simulink model "FinalProject_F24_thruster"  (R2023b)
settings: Solver=VariableStepAuto  StartTime=0.0  StopTime=720  FixedStep=.1  MaxStep=0.1  RelTol=1e-3
values from neighbouring files (symbols this model uses):
  h1 = I_s*ws1    [FinalProject_nonlinear_LVLH.m]
  h2 = I_s*ws2    [FinalProject_nonlinear_LVLH.m]
  h3 = I_s*ws3    [FinalProject_nonlinear_LVLH.m]
  hw_0 = [h1;h2;h3]    [FinalProject_nonlinear_LVLH.m]
  I_s =     [FinalProject_nonlinear_LVLH.m]
  I_T = diag([Ir;Ip;Iy])    [FinalProject_nonlinear_LVLH.m]
  K = lqr(A,B,Q,R)    [FinalProject_nonlinear_LVLH.m]
  omega_0 = [0;0;0]    [FinalProject_nonlinear_LVLH.m]
  omega_c = sqrt(mu/a^3)    [FinalProject_nonlinear_LVLH.m]
  q_0 = angle2quat(phi,theta,psi,'XYZ')'    [FinalProject_nonlinear_LVLH.m]
undefined symbols (not defined in the file or in its folder): E_des
libraries: sharedtransform x2
settings Model: Creator=Nathan.Collins  LastModifiedBy=Connor Emmons
settings OptimizationCC: ReuseModelBlockBuffer=off

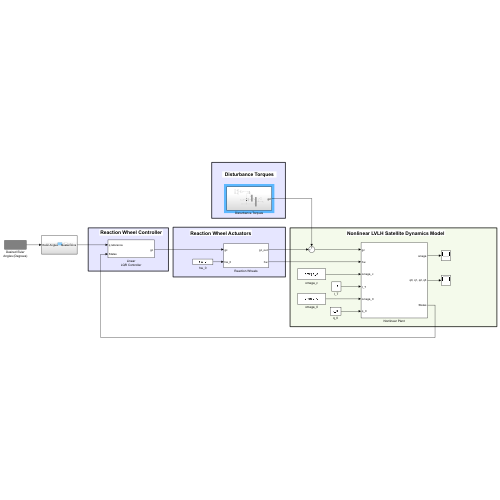
[thumbnail: Simulink's stored preview of the top-level diagram]
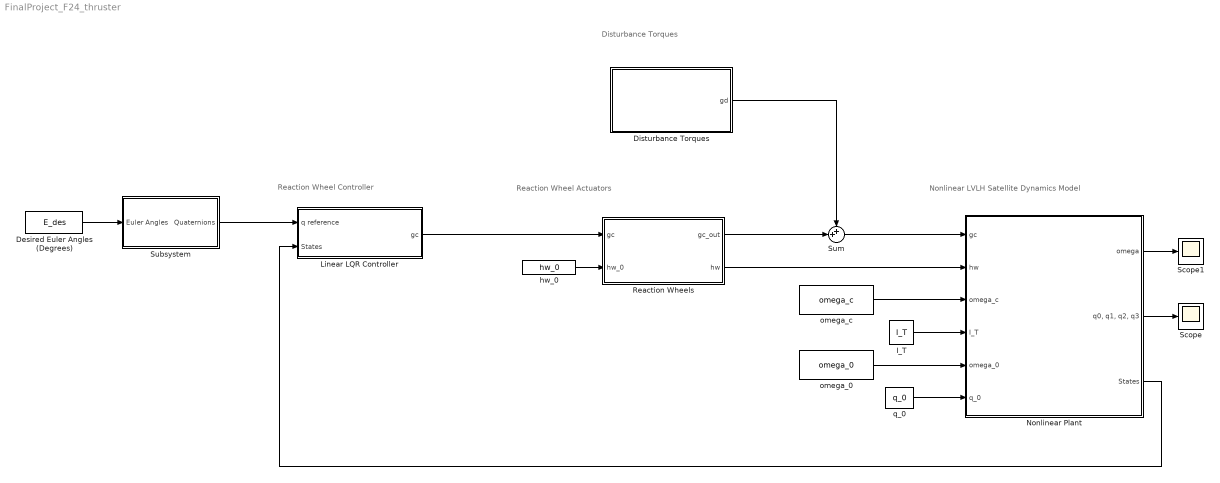
== system FinalProject_F24_thruster ==
  note: Reaction Wheel Actuators
  note: Nonlinear LVLH Satellite Dynamics Model
  note: Reaction Wheel Controller
  note: Disturbance Torques
  Desired Euler Angles (Degrees) : Constant  Value=E_des
  Disturbance Torques : Subsystem
  I_T : Constant  Value=I_T
  Linear LQR Controller : Subsystem
      settings: PortSchema="{\"entries\":[{\"content\":{\"sides\":[{\"content\":{\"connectorIds\":[\"Out1\"]},\"type\":\"ConnectorPlacement.EquallySpacedRectSide\",\"uuid\":\"ee26b0f2-a486-452c-b447-e59bb95ac0cf\"},{\"content\":{\"connectorIds\":[\"In1\",\"In2\"],\"side\":\"RIGHT\"},\"type\":\"ConnectorPlacement.EquallySpacedRectSide\",\"uuid\":\"56766a12-bb91-439a-8915-7afd5112c149\"},{\"content\":{\"connectorIds\":[],\"side\":\"TOP\"},\"type\":\"ConnectorPlacement.EquallySpacedRectSide\",\"uuid\":\"db65a026-f15d-443c-9f95-6ab7980aa8cf\"}]},\"type\":\"ConnectorPlacement.EquallySpacedConnector\",\"uuid\":\"3d1a91a6-4ad3-4b3e-bae7-10d191a9ffc1\"}],\"packageUris\":[\"http://schema.mathworks.com/mf0/Connector/R2020b\"],\"version\":\"1.0\"}"
  Nonlinear Plant : Subsystem
  Reaction Wheels : Subsystem
  Scope : Scope
  Scope1 : Scope
  Subsystem : Subsystem
  Sum : Sum  Inputs=++|
  hw_0 : Constant  Value=hw_0
  omega_0 : Constant  Value=omega_0
  omega_c : Constant  Value=omega_c
  q_0 : Constant  Value=q_0
  wires:
  Reaction Wheels/1(gc_out) -> Sum/2
  Reaction Wheels/2(hw) -> Nonlinear Plant/2(hw)
  omega_c/1 -> Nonlinear Plant/3(omega_c)
  I_T/1 -> Nonlinear Plant/4(I_T)
  hw_0/1 -> Reaction Wheels/2(hw_0)
  omega_0/1 -> Nonlinear Plant/5(omega_0)
  q_0/1 -> Nonlinear Plant/6(q_0)
  Linear LQR Controller/1(gc) -> Reaction Wheels/1(gc)
  Sum/1 -> Nonlinear Plant/1(gc)
  Disturbance Torques/1(gd) -> Sum/1
  Nonlinear Plant/2("q0, q1, q2, q3") -> Scope/1
  Nonlinear Plant/1(omega) -> Scope1/1
  Nonlinear Plant/3(States) -> Linear LQR Controller/2(States)
  Desired Euler Angles (Degrees)/1 -> Subsystem/1(Euler Angles)
  Subsystem/1(Quaternions) -> Linear LQR Controller/1(q reference)

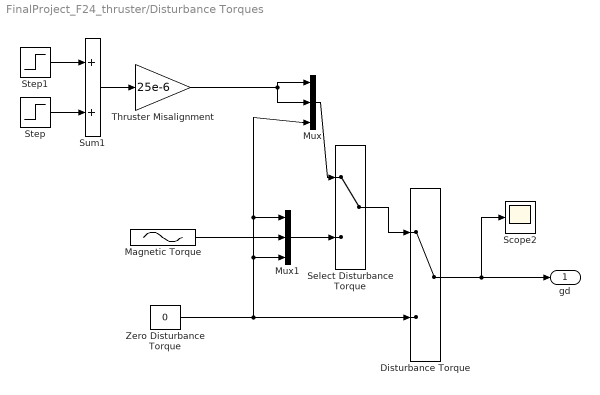
== system FinalProject_F24_thruster/Disturbance Torques ==
  Disturbance Torque : ManualSwitch
  Magnetic Torque : Sin  Amplitude=2e-6  Frequency=2*omega_c  SampleTime=0
  Mux : Mux  Inputs=3
  Mux1 : Mux  Inputs=3
  Scope2 : Scope
  Select Disturbance Torque : ManualSwitch
  Step : Step  Time=300  After=-1  SampleTime=0
  Step1 : Step  Time=0  SampleTime=0
  Sum1 : Sum
  Thruster Misalignment : Gain  Gain=25e-6
  Zero Disturbance Torque : Constant  Value=0
  gd : Outport
  wires:
  Thruster Misalignment/1 -> Mux/2, Mux/1
  Mux/1 -> Select Disturbance Torque/1
  Step1/1 -> Sum1/1
  Sum1/1 -> Thruster Misalignment/1
  Disturbance Torque/1 -> gd/1, Scope2/1
  Step/1 -> Sum1/2
  Zero Disturbance Torque/1 -> Mux/3, Mux1/1, Mux1/3, Disturbance Torque/2
  Mux1/1 -> Select Disturbance Torque/2
  Magnetic Torque/1 -> Mux1/2
  Select Disturbance Torque/1 -> Disturbance Torque/1

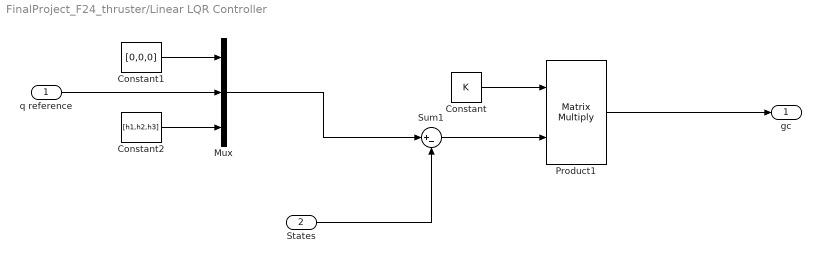
== system FinalProject_F24_thruster/Linear LQR Controller ==
  q reference : Inport
  States : Inport  Port=2
  Constant : Constant  Value=K
  Constant1 : Constant  Value=[0,0,0]
  Constant2 : Constant  Value=[h1,h2,h3]
  Mux : Mux  Inputs=3
  Product1 : Product  Multiplication=Matrix(*)
  Sum1 : Sum  Inputs=|+-
  gc : Outport
  wires:
  States/1 -> Sum1/2
  Product1/1 -> gc/1
  q reference/1 -> Mux/2
  Sum1/1 -> Product1/2
  Constant/1 -> Product1/1
  Constant1/1 -> Mux/1
  Mux/1 -> Sum1/1
  Constant2/1 -> Mux/3

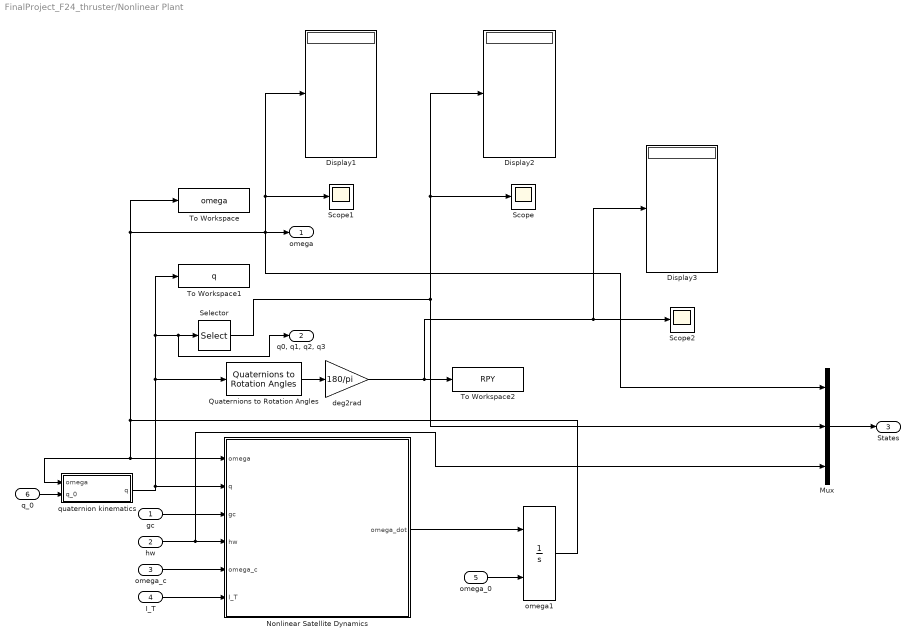
== system FinalProject_F24_thruster/Nonlinear Plant ==
  gc : Inport
  hw : Inport  Port=2
  omega_c : Inport  Port=3
  I_T : Inport  Port=4
  omega_0 : Inport  Port=5
  q_0 : Inport  Port=6
  Display1 : Display
  Display2 : Display
  Display3 : Display
  Mux : Mux  Inputs=3
  Nonlinear Satellite Dynamics : MATLAB Function  TreatAsAtomicUnit=on
  Quaternions to Rotation Angles : sharedtransform/Quaternions to Rotation Angles  rotationOrder=XYZ  aMode=aMode
  Scope : Scope
  Scope1 : Scope
  Scope2 : Scope
  Selector : Selector  InputPortWidth=4  IndexOptions=Index vector (dialog)  Indices=[2 3 4]  OutputSizes=1
  To Workspace : ToWorkspace  VariableName=omega  SaveFormat=Timeseries  SampleTime=-1
  To Workspace1 : ToWorkspace  VariableName=q  SaveFormat=Timeseries  SampleTime=-1
  To Workspace2 : ToWorkspace  VariableName=RPY  SaveFormat=Timeseries  SampleTime=-1
  deg2rad : Gain  Gain=180/pi
  omega1 : Integrator  InitialConditionSource=external
  quaternion kinematics : Subsystem
  omega : Outport
  "q0, q1, q2, q3" : Outport  Port=2
  States : Outport  Port=3
  wires:
  hw/1 -> Mux/3, Nonlinear Satellite Dynamics/4(hw)
  omega_0/1 -> omega1/2
  I_T/1 -> Nonlinear Satellite Dynamics/6(I_T)
  Nonlinear Satellite Dynamics/1(omega_dot) -> omega1/1
  gc/1 -> Nonlinear Satellite Dynamics/3(gc)
  omega_c/1 -> Nonlinear Satellite Dynamics/5(omega_c)
  quaternion kinematics/1(q) -> Quaternions to Rotation Angles/1, To Workspace1/1, "q0, q1, q2, q3"/1, Selector/1, Nonlinear Satellite Dynamics/2(q)
  omega1/1 -> quaternion kinematics/1(omega), Nonlinear Satellite Dynamics/1(omega), To Workspace/1, Mux/1, Display1/1, Scope1/1, omega/1
  Selector/1 -> Display2/1, Scope/1, Mux/2
  q_0/1 -> quaternion kinematics/2(q_0)
  Quaternions to Rotation Angles/1 -> deg2rad/1
  deg2rad/1 -> Display3/1, Scope2/1, To Workspace2/1
  Mux/1 -> States/1

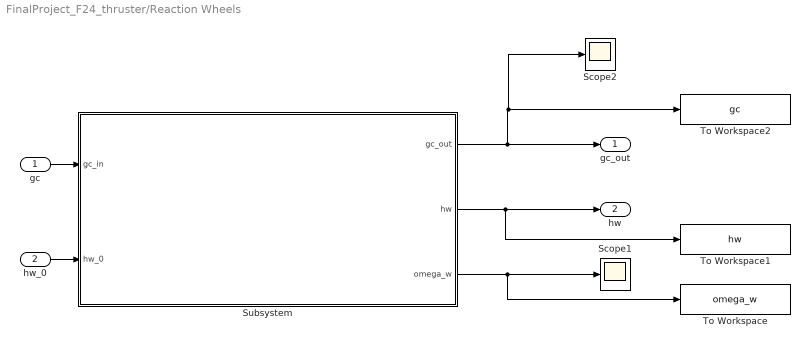
== system FinalProject_F24_thruster/Reaction Wheels ==
  gc : Inport
  hw_0 : Inport  Port=2
  Scope1 : Scope
  Scope2 : Scope
  Subsystem : Subsystem
  To Workspace : ToWorkspace  VariableName=omega_w  SaveFormat=Timeseries  SampleTime=-1
  To Workspace1 : ToWorkspace  VariableName=hw  SaveFormat=Timeseries  SampleTime=-1
  To Workspace2 : ToWorkspace  VariableName=gc  SaveFormat=Timeseries  SampleTime=-1
  gc_out : Outport
  hw : Outport  Port=2
  wires:
  Subsystem/1(gc_out) -> Scope2/1, To Workspace2/1, gc_out/1
  Subsystem/3(omega_w) -> To Workspace/1, Scope1/1
  Subsystem/2(hw) -> To Workspace1/1, hw/1
  gc/1 -> Subsystem/1(gc_in)
  hw_0/1 -> Subsystem/2(hw_0)

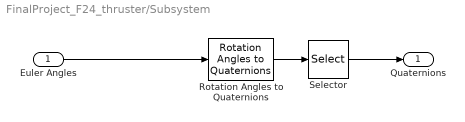
== system FinalProject_F24_thruster/Subsystem ==
  Euler Angles : Inport
  Rotation Angles to Quaternions : sharedtransform/Rotation Angles to Quaternions  rotationOrder=XYZ  aMode=aMode
  Selector : Selector  InputPortWidth=4  IndexOptions=Index vector (dialog)  Indices=[2 3 4]  OutputSizes=1
  Quaternions : Outport
  wires:
  Selector/1 -> Quaternions/1
  Rotation Angles to Quaternions/1 -> Selector/1
  Euler Angles/1 -> Rotation Angles to Quaternions/1

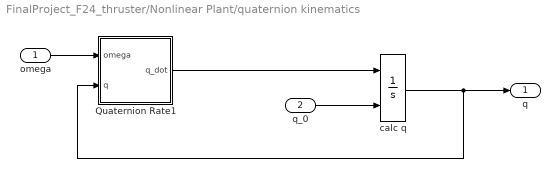
== system FinalProject_F24_thruster/Nonlinear Plant/quaternion kinematics ==
  omega : Inport
  q_0 : Inport  Port=2
  Quaternion Rate1 : Subsystem
  calc q : Integrator  InitialConditionSource=external
  q : Outport
  wires:
  q_0/1 -> calc q/2
  Quaternion Rate1/1(q_dot) -> calc q/1
  calc q/1 -> q/1, Quaternion Rate1/2(q)
  omega/1 -> Quaternion Rate1/1(omega)

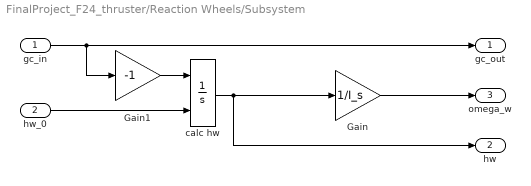
== system FinalProject_F24_thruster/Reaction Wheels/Subsystem ==
  gc_in : Inport
  hw_0 : Inport  Port=2
  Gain : Gain  Gain=1/I_s
  Gain1 : Gain  Gain=-1
  calc hw : Integrator  InitialConditionSource=external
  gc_out : Outport
  hw : Outport  Port=2
  omega_w : Outport  Port=3
  wires:
  calc hw/1 -> hw/1, Gain/1
  gc_in/1 -> gc_out/1, Gain1/1
  hw_0/1 -> calc hw/2
  Gain1/1 -> calc hw/1
  Gain/1 -> omega_w/1

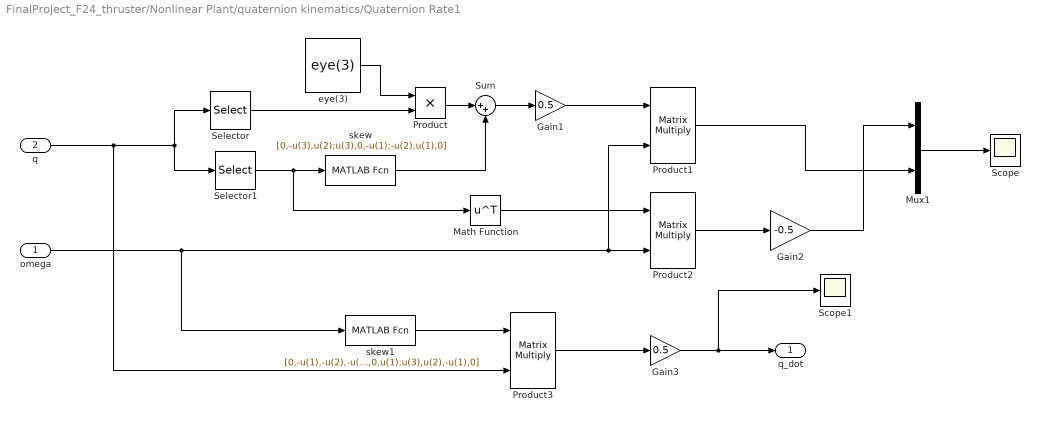
== system FinalProject_F24_thruster/Nonlinear Plant/quaternion kinematics/Quaternion Rate1 ==
  omega : Inport
  q : Inport  Port=2
  Gain1 : Gain  Gain=0.5
  Gain2 : Gain  Gain=-0.5
  Gain3 : Gain  Gain=0.5
  Math Function : Math  Operator=transpose
  Mux1 : Mux  Inputs=2
  Product : Product
  Product1 : Product  Multiplication=Matrix(*)
  Product2 : Product  Multiplication=Matrix(*)
  Product3 : Product  Multiplication=Matrix(*)
  Scope : Scope
  Scope1 : Scope
  Selector : Selector  InputPortWidth=4  IndexOptions=Index vector (dialog)  Indices=[1]  OutputSizes=1
  Selector1 : Selector  InputPortWidth=4  IndexOptions=Index vector (dialog)  Indices=[2 3 4]  OutputSizes=1
  Sum : Sum  Inputs=|++
  eye(3) : Constant  Value=eye(3)
  skew : MATLABFcn  MATLABFcn=[0,-u(3),u(2);u(3),0,-u(1);-u(2),u(1),0]  Output1D=off
  skew1 : MATLABFcn  MATLABFcn=[0,-u(1),-u(2),-u(3);u(1),0,u(3),-u(2);u(2),-u(3),0,u(1);u(3),u(2),-u(1),0]  Output1D=off
  q_dot : Outport
  wires:
  Product2/1 -> Gain2/1
  Product/1 -> Sum/1
  eye(3)/1 -> Product/1
  Math Function/1 -> Product2/1
  Gain2/1 -> Mux1/1
  Product1/1 -> Mux1/2
  Selector1/1 -> Math Function/1, skew/1
  skew/1 -> Sum/2
  Gain1/1 -> Product1/1
  Sum/1 -> Gain1/1
  omega/1 -> skew1/1, Product1/2, Product2/2
  Selector/1 -> Product/2
  q/1 -> Product3/2, Selector1/1, Selector/1
  skew1/1 -> Product3/1
  Product3/1 -> Gain3/1
  Gain3/1 -> Scope1/1, q_dot/1
  Mux1/1 -> Scope/1

== matlab function FinalProject_F24_thruster/Nonlinear Plant/Nonlinear Satellite Dynamics ==
  data: omega input; q input; gc input; hw input; omega_dot output; omega_c input; I_T input
function omega_dot = fcn(omega,q,gc,hw,omega_c,I_T)

q0 = q(1);
q1 = q(2);
q2 = q(3);
q3 = q(4);

Q1 = [2*q0^2 - 1 + 2*q1^2;...
    2*q1*q2 - 2*q0*q3;...
    2*q1*q3 + 2*q0*q2];

Q2 = [2*q1*q2 + 2*q0*q3;...
    2*q0^2 - 1 + 2*q2^2;...
    2*q2*q3 - 2*q0*q1];

Q3 = [2*q1*q3 - 2*q0*q2;...
    2*q2*q3 + 2*q0*q1;...
    2*q0^2 - 1 + 2*q3^2];

Q_po = [Q1,Q2,Q3];

w_c = [0;-omega_c;0];

invI_T = I_T^-1;

w = omega + Q_po*w_c;

Q_po_dot = -skew(w)*Q_po + Q_po*skew(w_c);

cb = Q_po*[0;0;1];

omega_dot = invI_T*(-I_T*Q_po_dot*w_c - cross(w,I_T*w + hw) + gc + 3*omega_c^2*cross(cb,I_T*cb));
end

function a_x = skew(a)

a_x = [0,-a(3),a(2);...
    a(3),0,-a(1);...
    -a(2),a(1),0];
end
